simulink model "optimiser"  (Simulink 8.1)
settings: Solver=ode45  StartTime=0.0  StopTime=10.0  RelTol=1e-3
values from neighbouring files (symbols this model uses):
  P = lmivar(1,[2 1])    [hybrid_linear_setup.m]
  x0 = [1;1]    [hybrid_linear_setup.m]
undefined symbols (not defined in the file or in its folder): A, B, K, x1
libraries: dspmtrx3 x3, simulink x2, Numerical x2, Is_equal_scalar x1, goal x1
settings Model: Creator=dejanira  LastModifiedBy=dejanira
settings DataIOCC: SignalLoggingSaveFormat=Dataset
settings OptimizationCC: ExpressionDepthLimit=128
settings DebuggingCC: FcnCallInpInsideContextMsg=EnableAllAsError
settings GRTTargetCC: CombineOutputUpdateFcns=on  GRTInterface=off

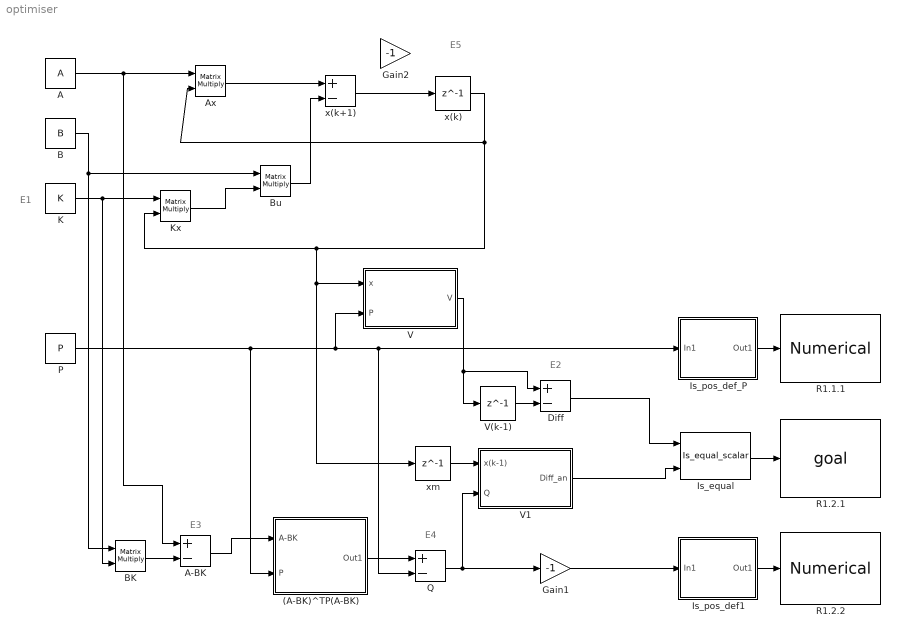
== system optimiser ==
  note: E1
  note: E2
  note: E3
  note: E4
  note: E5
  (A-BK)^TP(A-BK) : Subsystem  mask(Quadratic){}
  A : Constant  Value=A  VectorParams1D=off
  A-BK : Sum  Inputs=+-
  Ax : Product  Multiplication=Matrix(*)
  B : Constant  Value=B  VectorParams1D=off
  BK : Product  Multiplication=Matrix(*)
  Bu : Product  Multiplication=Matrix(*)
  Diff : Sum  Inputs=+-
  Gain1 : Gain  Gain=-1
  Gain2 : Gain  Gain=-1
  Is_equal : Is_equal_scalar/Is_equal_scalar  SystemSampleTime=-1
  Is_pos_def1 : Subsystem  TreatAsAtomicUnit=on  mask(Is_pos_def){}
      mask Display:
      | port_label('input',1,'matrix')
      | port_label('output',1,'T/F')
  Is_pos_def_P : Subsystem  TreatAsAtomicUnit=on  mask(Is_pos_def){}
      mask Display:
      | port_label('input',1,'matrix')
      | port_label('output',1,'T/F')
  K : Constant  Value=K  VectorParams1D=off
  Kx : Product  Multiplication=Matrix(*)
  P : Constant  Value=P  VectorParams1D=off
  Q : Sum  Inputs=+-
  R1.1.1 : Numerical/Numerical  SystemSampleTime=-1
  R1.2.1 : goal/goal  SystemSampleTime=-1
  R1.2.2 : Numerical/Numerical  SystemSampleTime=-1
  V : Subsystem  mask(Quadratic){}
  V(k-1) : Delay  DelayLength=1  InitialCondition=x0'*P*x0  SampleTime=0.1
  V1 : Subsystem  mask(Quadratic){}
  x(k) : Delay  DelayLength=1  InitialCondition=x1  SampleTime=0.1
  x(k+1) : Sum  Inputs=+-
  xm : Delay  DelayLength=1  InitialCondition=x0  SampleTime=0.1
  wires:
  K/1 -> Kx/1, BK/2
  V/1(V) -> V(k-1)/1, Diff/1
  Diff/1 -> Is_equal/1
  Is_pos_def_P/1(Out1) -> R1.1.1/1
  Is_pos_def1/1(Out1) -> R1.2.2/1
  A-BK/1 -> (A-BK)^TP(A-BK)/1(A-BK)
  Q/1 -> V1/2(Q), Gain1/1
  xm/1 -> V1/1(x(k-1))
  V1/1(Diff_an) -> Is_equal/2
  Is_equal/1 -> R1.2.1/1
  x(k)/1 -> Ax/2, xm/1, V/1(x), Kx/2
  A/1 -> A-BK/1, Ax/1
  Kx/1 -> Bu/2
  Bu/1 -> x(k+1)/2
  Ax/1 -> x(k+1)/1
  B/1 -> BK/1, Bu/1
  (A-BK)^TP(A-BK)/1(Out1) -> Q/1
  P/1 -> Q/2, Is_pos_def_P/1(In1), V/2(P), (A-BK)^TP(A-BK)/2(P)
  BK/1 -> A-BK/2
  x(k+1)/1 -> x(k)/1
  Gain1/1 -> Is_pos_def1/1(In1)
  V(k-1)/1 -> Diff/2

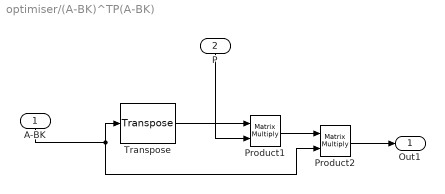
== system optimiser/(A-BK)^TP(A-BK) ==
  A-BK : Inport
  P : Inport  Port=2
  Product1 : Product  Multiplication=Matrix(*)
  Product2 : Product  Multiplication=Matrix(*)
  Transpose : dspmtrx3/Transpose  Hermitian=off  overflowFlag=off
  Out1 : Outport
  wires:
  Product1/1 -> Product2/1
  Product2/1 -> Out1/1
  A-BK/1 -> Transpose/1, Product2/2
  P/1 -> Product1/2
  Transpose/1 -> Product1/1

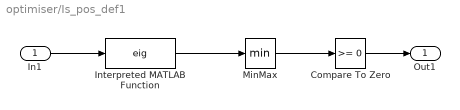
== system optimiser/Is_pos_def1 ==
  In1 : Inport
  Compare To Zero : simulink/Logic and Bit Operations/Compare To Zero  relop=>=  OutDataTypeStr=boolean
  Interpreted MATLAB Function : MATLABFcn  MATLABFcn=eig
  MinMax : MinMax
  Out1 : Outport
  wires:
  Interpreted MATLAB Function/1 -> MinMax/1
  Compare To Zero/1 -> Out1/1
  In1/1 -> Interpreted MATLAB Function/1
  MinMax/1 -> Compare To Zero/1

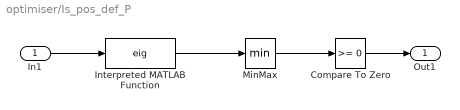
== system optimiser/Is_pos_def_P ==
  In1 : Inport
  Compare To Zero : simulink/Logic and Bit Operations/Compare To Zero  relop=>=  OutDataTypeStr=boolean
  Interpreted MATLAB Function : MATLABFcn  MATLABFcn=eig
  MinMax : MinMax
  Out1 : Outport
  wires:
  Interpreted MATLAB Function/1 -> MinMax/1
  Compare To Zero/1 -> Out1/1
  In1/1 -> Interpreted MATLAB Function/1
  MinMax/1 -> Compare To Zero/1

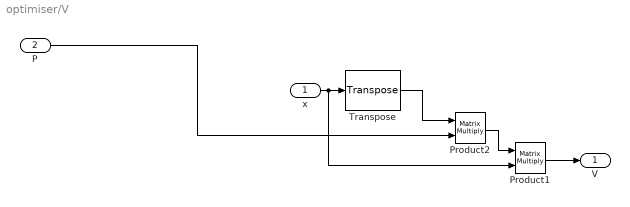
== system optimiser/V ==
  x : Inport
  P : Inport  Port=2
  Product1 : Product  Multiplication=Matrix(*)
  Product2 : Product  Multiplication=Matrix(*)
  Transpose : dspmtrx3/Transpose  Hermitian=off  overflowFlag=off
  V : Outport
  wires:
  P/1 -> Product2/2
  x/1 -> Product1/2, Transpose/1
  Product1/1 -> V/1
  Product2/1 -> Product1/1
  Transpose/1 -> Product2/1

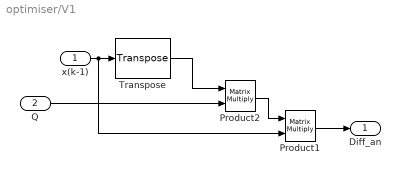
== system optimiser/V1 ==
  x(k-1) : Inport
  Q : Inport  Port=2
  Product1 : Product  Multiplication=Matrix(*)
  Product2 : Product  Multiplication=Matrix(*)
  Transpose : dspmtrx3/Transpose  Hermitian=off  overflowFlag=off
  Diff_an : Outport
  wires:
  Q/1 -> Product2/2
  x(k-1)/1 -> Product1/2, Transpose/1
  Product1/1 -> Diff_an/1
  Product2/1 -> Product1/1
  Transpose/1 -> Product2/1
